simulink model "batchintro"  (R2018a)
settings: Solver=VariableStepAuto  StartTime=0.0  StopTime=15  RelTol=1e-3
settings Model: Creator=kudva  LastModifiedBy=kudva

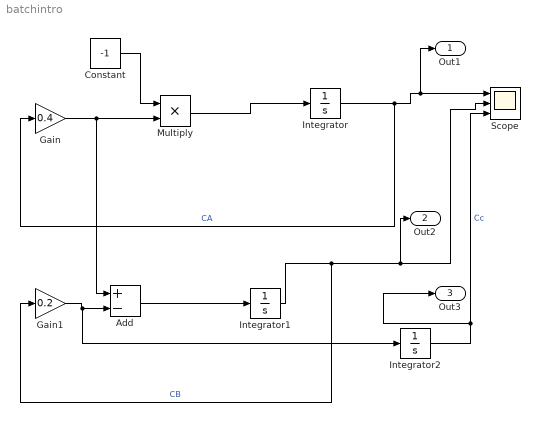
== system batchintro ==
  Add : Sum  Inputs=+-
  Constant : Constant  Value=-1
  Gain : Gain  Gain=0.4
  Gain1 : Gain  Gain=0.2
  Integrator : Integrator  InitialCondition=5
  Integrator1 : Integrator
  Integrator2 : Integrator
  Multiply : Product
  Scope : Scope  NumInputPorts=3
  Out1 : Outport
  Out2 : Outport  Port=2
  Out3 : Outport  Port=3
  wires:
  Gain/1 -> Add/1, Multiply/2
  Constant/1 -> Multiply/1
  Multiply/1 -> Integrator/1
  Integrator/1 -> Gain/1, Out1/1, Scope/1  "CA"
  Gain1/1 -> Integrator2/1, Add/2
  Add/1 -> Integrator1/1
  Integrator1/1 -> Gain1/1, Out2/1, Scope/2  "CB"
  Integrator2/1 -> Out3/1, Scope/3  "Cc"
